simulink model "ac_braxykyklwma"  (R2022a)
settings: Solver=ode23tb  StartTime=0.0  StopTime=3  MaxStep=1e-5  RelTol=1e-3
libraries: spsRMSLib x2, spsControlledVoltageSourceLib x1, simulink x1, spsCurrentMeasurementLib x1, spsPowerLib x1, spsVoltageMeasurementLib x1, spsSaturableTransformerLib x1, spspowerguiLib x1
settings Model: Creator=User  LastModifiedBy=User

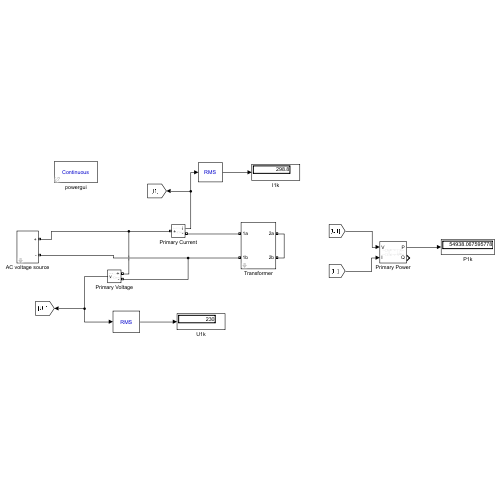
[thumbnail: Simulink's stored preview of the top-level diagram]
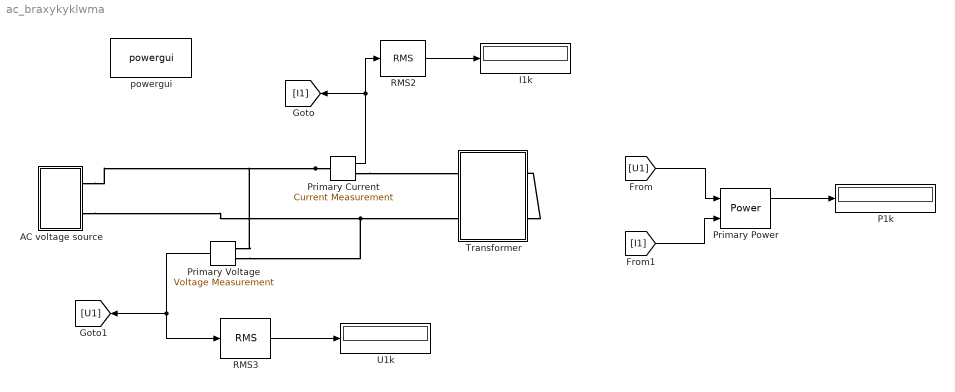
== system ac_braxykyklwma ==
  AC voltage source : Subsystem  mask{Vrms=230}
  I1k : Display
  P1k : Display
  Primary Current : spsCurrentMeasurementLib/Current Measurement  PhasorSimulation=off  OutputType=Complex  PSBequivalent=0
  Primary Power : spsPowerLib/Power  Freq=50  Vinit=[0, 0]  Iinit=[0, 0]  Ts=0
      settings: SourceProductBaseCode=PS
  Primary Voltage : spsVoltageMeasurementLib/Voltage Measurement  PhasorSimulation=off  OutputType=Complex  PSBequivalent=0
  RMS2 : spsRMSLib/RMS  TrueRMS=on  Freq=50  RMSInit=0  Ts=0
  RMS3 : spsRMSLib/RMS  TrueRMS=on  Freq=50  RMSInit=0  Ts=0
  Transformer : Subsystem  mask{PN=4, U1N=230, U2N=115}
      mask prompts: PN "PN (kVA)"; U1N "U1N (V)"; U2N "U2N (V)"
  U1k : Display
  powergui : spspowerguiLib/powergui  Priority=1  SimulationMode=Continuous  SampleTime=50e-6  frequency=60  Iterations=50  frequencyindice=0  Pbase=100e6  ErrMax=1e-4  UnitsV=kV  UnitsW=MW  buscounter=0  FunctionMessages=off  echomessages=off  EnableUseOfTLC=off  CurrentSourceSwitches=off  DisableSnubberDevices=off  DisableRonSwitches=off  DisableVfSwitches=off  DisplayEquations=off  AutomaticDiscreteSolvers=off  SolverType=Tustin/Backward Euler (TBE)  Interpol=off  ExternalGateDelay=off  methode=off  Ts=100  x0status=blocks  SPID=on  SwTol=0  HookPort=off  NonlinearTolerance=1e-4  nMaxIteration=100  ContinueOnMaxIteration=off  RestoreLinks=warning  ResistiveCurrentMeasurement=off  Frange=[0:2:500]  Ylog=off  Xlog=on  ShowGrid=off  save=off  variable=ZData  structure=0  ZoomFFT=off  StartTime=0.0  cycles=1  DisplayStyle=1  fundamental=60  FreqAxis=off  MaxFrequency=1000  frequencyindicesteady=1  RmsSteady=1  display=off
  wires:
  Primary Power/1 -> P1k/1
  Primary Voltage/1 -> [U1], RMS3/1
  [U1] -> Primary Power/1
  RMS3/1 -> U1k/1
  Primary Current/1 -> RMS2/1, [I1]
  RMS2/1 -> I1k/1
  [I1] -> Primary Power/2
  connections:
  Primary Voltage/LConn2 -- AC voltage source/RConn2 -- Transformer/LConn2
  Primary Current/LConn1 -- AC voltage source/RConn1 -- Primary Voltage/LConn1
  Primary Current/RConn1 -- Transformer/LConn1
  Transformer/RConn2 -- Transformer/RConn1

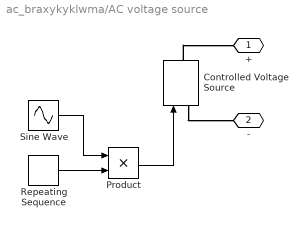
== system ac_braxykyklwma/AC voltage source ==
  Controlled Voltage Source : spsControlledVoltageSourceLib/Controlled Voltage Source  Initialize=on  Source_Type=AC  Amplitude=0  Phase=0  Frequency=50  Measurements=Voltage
  Product : Product
  Repeating Sequence : simulink/Sources/Repeating Sequence  rep_seq_t=[0 0.5 1000]  rep_seq_y=[0 Vrms Vrms]
  Sine Wave : Sin  Amplitude=sqrt(2)  Frequency=100*pi  SampleTime=0
  + : PMIOPort  Side=Right
  - : PMIOPort  Port=2  Side=Right
  wires:
  Product/1 -> Controlled Voltage Source/1
  Sine Wave/1 -> Product/1
  Repeating Sequence/1 -> Product/2
  connections:
  Controlled Voltage Source/LConn1 -- -/RConn1
  Controlled Voltage Source/RConn1 -- +/RConn1

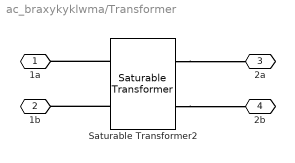
== system ac_braxykyklwma/Transformer ==
  Saturable Transformer2 : spsSaturableTransformerLib/Saturable Transformer  ThreeWindings=off  Hysteresis=off  DataFile='hysteresis.mat'  Measurements=None  UNITS=pu  NominalPower=[4e3 50]  Winding1=[230 0.022273 0.015903]  Winding2=[122 0.024298 0.019083]  Winding3=[3.15e+05 0.00245 0.098001]  Saturation=[0 0;0.031714 0.76205;0.037813 0.86926;0.045538 0.94653;0.060175 1.0141;0.080911 1.0624;0.14637 1.159]  CoreLoss=35.539  BreakLoop=off  DiscreteSolver=Trapezoidal iterative  DataType=off  InitialFlux=0  TransfoNumber=1
      settings: SourceProductBaseCode=PS
  1a : PMIOPort  Side=Left
  1b : PMIOPort  Port=2  Side=Left
  2a : PMIOPort  Port=3  Side=Right
  2b : PMIOPort  Port=4  Side=Right
  connections:
  Saturable Transformer2/RConn2 -- 2b/RConn1
  Saturable Transformer2/LConn1 -- 1a/RConn1
  Saturable Transformer2/RConn1 -- 2a/RConn1
  Saturable Transformer2/LConn2 -- 1b/RConn1
